simulink model "WholeModelPIDFeedFowardDigital"  (R2020b)
settings: Solver=ode45  StartTime=0.0  StopTime=5  RelTol=1e-3
values from neighbouring files (symbols this model uses):
  Ts = T2    (= 0.01)    [PIDAntiWindupDigital.m]    (also in PIDDigital.m = 0.001; StateSpaceControllerNominalCont.m = 0.001; StateSpaceControllerNominalDigital.m = 0.001; StateSpaceControllerNominalDirectDigital.m = 0.05)
undefined symbols (not defined in the file or in its folder): DiscIntNeverNeededParam, rpm2degs, rpm2rads
libraries: simulink x1
settings Model: Creator=umberto  LastModifiedBy=umbe

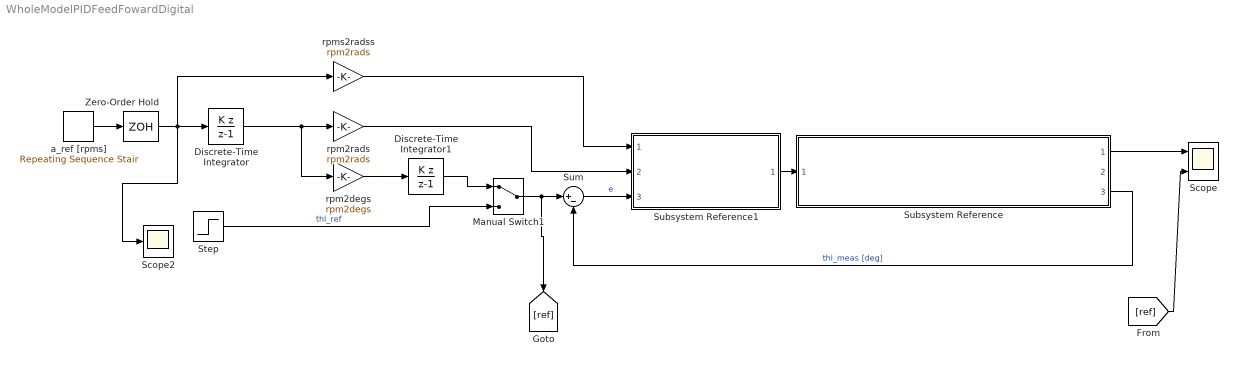
== system WholeModelPIDFeedFowardDigital ==
  Discrete-Time Integrator : DiscreteIntegrator  IntegratorMethod=Accumulation: Backward Euler  gainval=Ts  SampleTime=Ts  ICPrevOutput=DiscIntNeverNeededParam  ICPrevScaledInput=DiscIntNeverNeededParam
  Discrete-Time Integrator1 : DiscreteIntegrator  IntegratorMethod=Accumulation: Backward Euler  gainval=Ts  SampleTime=Ts  ICPrevOutput=DiscIntNeverNeededParam  ICPrevScaledInput=DiscIntNeverNeededParam
  Manual Switch1 : ManualSwitch
  Scope : Scope  NumInputPorts=2
  Scope2 : Scope
  Step : Step  Time=0  After=360  SampleTime=0
  Subsystem Reference : Subsystem  ReferencedSubsystem=DCServoMotor_SubSystem
  Subsystem Reference1 : Subsystem  ReferencedSubsystem=PIDFeedFowardDigital_SubSystem
  Sum : Sum  Inputs=|+-
  Zero-Order Hold : ZeroOrderHold  SampleTime=Ts
  a_ref [rpms] : simulink/Sources/Repeating Sequence Stair  OutValues=[900 0 -900 -900 0 900].'  tsamp=0.5  OutMin=[]  OutMax=[]  OutDataTypeStr=double  OutputDataTypeScalingMode=double  OutDataType=fixdt(0,8)  ConRadixGroup=Best Precision: Vector-wise  OutScaling=2^-12
  rpm2degs : Gain  Gain=rpm2degs
  rpm2rads : Gain  Gain=rpm2rads
  rpms2radss : Gain  Gain=rpm2rads
  wires:
  Subsystem Reference/3 -> Sum/2  "thl_meas [deg]"
  Step/1 -> Manual Switch1/2  "thl_ref"
  Subsystem Reference/1 -> Scope/1
  Sum/1 -> Subsystem Reference1/3  "e"
  [ref] -> Scope/2
  Subsystem Reference1/1 -> Subsystem Reference/1
  rpms2radss/1 -> Subsystem Reference1/1
  rpm2rads/1 -> Subsystem Reference1/2
  rpm2degs/1 -> Discrete-Time Integrator1/1
  a_ref [rpms]/1 -> Zero-Order Hold/1
  Discrete-Time Integrator1/1 -> Manual Switch1/1
  Discrete-Time Integrator/1 -> rpm2degs/1, rpm2rads/1
  Manual Switch1/1 -> [ref], Sum/1
  Zero-Order Hold/1 -> Scope2/1, Discrete-Time Integrator/1, rpms2radss/1
